simulink model "robot_planare"  (Simulink 7.2)
settings: Solver=ode45  StartTime=0.0  StopTime=Tf  FixedStep=1e-3  RelTol=1e-5
values from neighbouring files (symbols this model uses):
  beta10 = beta1r(1)    [s_robot_planare.m]
  beta20 = beta2r(1)    [s_robot_planare.m]
  kd1 = h*2*a    [s_robot_planare.m]
  kd2 = h*2*a    [s_robot_planare.m]
  kp1 = h*2*a^2    [s_robot_planare.m]
  kp2 = h*2*a^2    [s_robot_planare.m]
  Lb1 = 0.3    [s_robot_planare.m]
  Lb2 = 0.4    [s_robot_planare.m]
  tauf = .05    (= 0.05)    [s_robot_planare.m]
libraries: simulink_extras x4
settings Model: Creator=prof. G. Celentano  LastModifiedBy=gle  ExtModeTrigMode=oneshot  ExtModeArmWhenConnect=off
settings DataIOCC: LimitDataPoints=off  SignalLoggingName=sigsOut
settings OptimizationCC: BooleanDataType=off  InitFltsAndDblsToZero=on
settings DebuggingCC: SaveWithParameterizedLinksMsg=none  SignalResolutionControl=TryResolveAllWithWarning  SolverPrmCheckMsg=none  MultiTaskDSMMsg=warning  MultiTaskCondExecSysMsg=none  StrictBusMsg=None
settings HardwareCC: TargetUnknown=on
settings RTWCC: IncludeERTFirstTime=on
settings GRTTargetCC: TargetFcnLib=ansi_tfl_tmw.mat

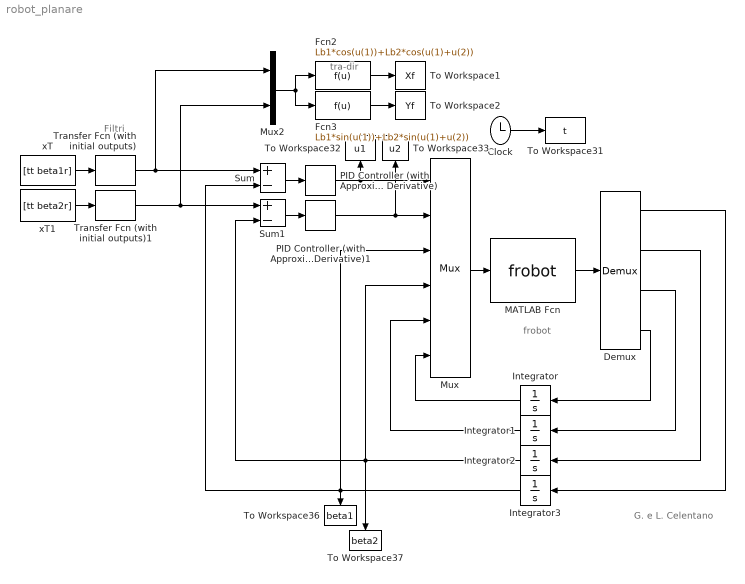
== system robot_planare ==
  note: frobot
  note: G. e L. Celentano
  note: Filtri
  note: tra-dir
  Clock : Clock
      settings: Decimation=10
  Demux : Demux
  Fcn2 : Fcn  Expr=Lb1*cos(u(1))+Lb2*cos(u(1)+u(2))
  Fcn3 : Fcn  Expr=Lb1*sin(u(1))+Lb2*sin(u(1)+u(2))
  Integrator : Integrator  Orientation=left
  Integrator1 : Integrator  Orientation=left
  Integrator2 : Integrator  Orientation=left  InitialCondition=beta20
  Integrator3 : Integrator  Orientation=left  InitialCondition=beta10
  MATLAB Fcn : MATLABFcn  MATLABFcn=frobot  OutputDimensions=4
  Mux : Mux  Inputs=6
  Mux2 : Mux  Inputs=[1 1]
  PID Controller (with Approximate Derivative) : simulink_extras/Additional Linear/PID Controller (with Approximate Derivative)  SystemSampleTime=-1  P=kp1  I=0  D=kd1  N=10
  PID Controller (with Approximate Derivative)1 : simulink_extras/Additional Linear/PID Controller (with Approximate Derivative)  SystemSampleTime=-1  P=kp2  I=0  D=kd2  N=10
  Sum : Sum  Inputs=+-  OutDataType=sfix(16)  OutScaling=2^0  SaturateOnIntegerOverflow=on  InputSameDT=on  OutDataTypeStr=Inherit: Same as first input
  Sum1 : Sum  Inputs=+-  OutDataType=sfix(16)  OutScaling=2^0  SaturateOnIntegerOverflow=on  InputSameDT=on  OutDataTypeStr=Inherit: Same as first input
  To Workspace1 : ToWorkspace  VariableName=Xf  SampleTime=-1  SaveFormat=Array
  To Workspace2 : ToWorkspace  VariableName=Yf  SampleTime=-1  SaveFormat=Array
  To Workspace31 : ToWorkspace  VariableName=t  SampleTime=-1  SaveFormat=Array
  To Workspace32 : ToWorkspace  VariableName=u1  SampleTime=-1  SaveFormat=Array
      settings: Orientation=up
  To Workspace33 : ToWorkspace  VariableName=u2  SampleTime=-1  SaveFormat=Array
      settings: Orientation=up
  To Workspace36 : ToWorkspace  VariableName=beta1  SampleTime=-1  SaveFormat=Array
      settings: Orientation=down
  To Workspace37 : ToWorkspace  VariableName=beta2  SampleTime=-1  SaveFormat=Array
      settings: Orientation=down
  Transfer Fcn (with initial outputs) : simulink_extras/Additional Linear/Transfer Fcn (with initial outputs)  SystemSampleTime=-1  N=[1]  D="[tauf  1]"  Y0=beta10  U0=0
  Transfer Fcn (with initial outputs)1 : simulink_extras/Additional Linear/Transfer Fcn (with initial outputs)  SystemSampleTime=-1  N=[1]  D="[tauf  1]"  Y0=beta20  U0=0
  xT : FromWorkspace  VariableName="[tt  beta1r]"  SampleTime=0
  xT1 : FromWorkspace  VariableName="[tt  beta2r]"  SampleTime=0
  wires:
  Clock/1 -> To Workspace31/1
  Mux/1 -> MATLAB Fcn/1
  MATLAB Fcn/1 -> Demux/1
  Demux/4 -> Integrator/1
  Demux/3 -> Integrator1/1
  Demux/1 -> Integrator3/1
  Demux/2 -> Integrator2/1
  Integrator3/1 -> Sum/2, Mux/3, To Workspace36/1
  PID Controller (with Approximate Derivative)/1 -> To Workspace32/1, Mux/1
  Sum/1 -> PID Controller (with Approximate Derivative)/1
  Sum1/1 -> PID Controller (with Approximate Derivative)1/1
  PID Controller (with Approximate Derivative)1/1 -> Mux/2, To Workspace33/1
  Integrator2/1 -> Mux/4, Sum1/2, To Workspace37/1
  Integrator/1 -> Mux/6
  Integrator1/1 -> Mux/5
  xT/1 -> Transfer Fcn (with initial outputs)/1
  xT1/1 -> Transfer Fcn (with initial outputs)1/1
  Transfer Fcn (with initial outputs)/1 -> Sum/1, Mux2/1
  Transfer Fcn (with initial outputs)1/1 -> Sum1/1, Mux2/2
  Mux2/1 -> Fcn2/1, Fcn3/1
  Fcn2/1 -> To Workspace1/1
  Fcn3/1 -> To Workspace2/1
